simulink model "motor_simscapepump"  (R2014a)
settings: Solver=ode15s  StartTime=0.0  StopTime=1  MaxStep=0.2  RelTol=1e-4
undefined symbols (not defined in the file): D1, Delta
libraries: powerlib x6, fl_lib x4, nesl_utility x2, sh_lib x1
settings Model: Creator=scastro  LastModifiedBy=cosorio
settings DataIOCC: SaveOutput=off  SaveTime=off
settings DebuggingCC: UnderspecifiedInitializationDetection=Classic  MultiTaskDSMMsg=warning  MultiTaskCondExecSysMsg=none
settings RTWCC: IncludeERTFirstTime=on

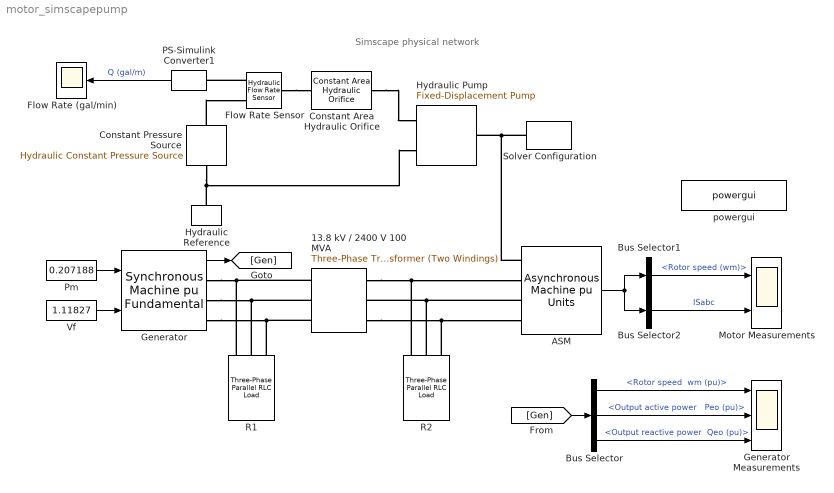
== system motor_simscapepump ==
  note: Simscape physical network
  13.8 kV / 2400 V 100 MVA : powerlib/Elements/Three-Phase Transformer (Two Windings)  Winding1Connection=Yg  UNITS=pu  NominalPower=[ 100e6 , 60 ]  Winding1=[ 13800 , 0.002 , 0.08 ]  Winding2Connection=Delta (D1)  Winding2=[ 2400 , 0.002 , 0.08 ]  SetSaturation=off  Rm=500  Lm=500  Saturation=[ 0,0 ; 0.0024,1.2 ; 1.0,1.52 ]  Hysteresis=off  DataFile='hysteresis'  SetInitialFlux=off  InitialFluxes=[ 0.8 , -0.8 , 0.7 ]  Measurements=None  MoreParameters=off  BreakLoop=off  DataType=off  TransfoNumber=1
  ASM : powerlib/Machines/Asynchronous Machine pu Units  PresetModel=No  MechanicalLoad=Mechanical rotational port  ShowDetailedParameters=on  RotorType=Squirrel-cage  ReferenceFrame=Rotor  Units=pu  MeasurementBus=off  NominalParameters=[10e6 2400 60]  Stator=[0.01965 0.0397]  Rotor=[0.01909 0.0397]  Cage1=[0.01909 0.0397]  Cage2=[0.01909 0.0397]  Lm=1.354  Mechanical=[0.09526 0.05479 2]  PolePairs=2  InitialConditions=[0.00133172 0 0.711213 0.711213 0.711213 -114.92 125.08 5.08024]  SimulateSaturation=off  Saturation="[0.212,0.4201,0.8125,1.0979,1.4799,2.2457,3.2586,4.5763,6.4763 ;   0.5,0.7,0.9,1,1.1,1.2 ,1.3,1.4,1.5]"  LoadFlowParameters=640000  TsPowergui=0  TsBlock=-1  IterativeModel=Trapezoidal non iterative  Pmec=25e6
      settings: AttributesFormatString=%<NominalParameters>
  Bus Selector : BusSelector  OutputSignals="Mechanical.Rotor speed  wm (pu),Output active power   Peo (pu),Output reactive power  Qeo (pu)"
  Bus Selector1 : BusSelector  OutputSignals=Mechanical.Rotor speed (wm)
  Bus Selector2 : BusSelector  OutputSignals=Stator measurements.Stator current is_a (pu),Stator measurements.Stator current is_b (pu),Stator measurements.Stator current is_c (pu)  OutputAsBus=on
  Constant Pressure Source : fl_lib/Hydraulic/Hydraulic Sources/Hydraulic Constant Pressure Source  commanded_pressure=50e5 Pa
      settings: AttributesFormatString=P = %<commanded_pressure> Pa
  Constant Area Hydraulic Orifice : fl_lib/Hydraulic/Hydraulic Elements/Constant Area Hydraulic Orifice  area=5e-4 m^2  C_d=0.7  Re_cr=12  D_h=0.0113 m  p_cr=1 Pa  q_specify=off  q_priority=High  q=1 m^3/s  p_specify=off  p_priority=High  p=0 Pa
  Flow Rate (gal/min) : Scope
      settings: YMin=0  YMax=300  SaveName=ScopeData4
  Flow Rate Sensor : fl_lib/Hydraulic/Hydraulic Sensors/Hydraulic Flow Rate Sensor
  Generator : powerlib/Machines/Synchronous Machine pu Fundamental  PresetModel=No  MechanicalLoad=Mechanical power Pm  ShowDetailedParameters=on  RotorType=Salient-pole  Units=per unit fundamental parameters  MeasurementBus=off  NominalParameters="[ 100E6  13800   60]"  Stator="[ 2.85E-03  0.114  1.19  0.36 ]"  Field="[ 5.79E-04  0.114]"  Dampers2=[0.0652, 0.5134, 0.0287, 0.2553, 7.765e-3, 0.9167 ]  Dampers1="[ 1.17E-02  0.182  1.97E-02  0.384 ]"  Mechanical=[ 3.7 0 2 ]  PolePairs=2  InitialConditions=[0 -84.5996 0.22005 0.22005 0.22005 -19.793 -139.793 100.207 1.11827]  SetSaturation=off  Saturation=[0.6404,0.7127,0.8441,0.9214,0.9956,1.082,1.19,1.316,1.457;0.7,0.7698,0.8872,0.9466,0.9969,1.046,1.1,1.151,1.201]  LoadFlowParameters=[2 75000000 13800 0 25000000]  TsPowergui=0  TsBlock=-1  IterativeModel=Trapezoidal non iterative  BusType=PQ  Pref=75e6  Qref=25e6  Qmin=-inf  Qmax=inf  PLF=0  QLF=0
      settings: AttributesFormatString=%<NominalParameters>
  Generator Measurements : Scope  NumInputPorts=3
      settings: YMin=0~0~0  YMax=1.5~1~1
  Hydraulic Pump : sh_lib/Pumps and Motors/Fixed-Displacement Pump  D=7.5e-5 m^3/rad  efficiency_vol=0.9  efficiency_tot=0.8  pr_nominal=100e5 Pa  w_nominal=60*2*pi rad/s  visc_nominal=18 cSt  dens_nominal=900 kg/m^3  k_leak=1e-11 m^3/s/Pa  efficiency_mech=0.7
  Hydraulic Reference : fl_lib/Hydraulic/Hydraulic Elements/Hydraulic Reference
  Motor Measurements : Scope  NumInputPorts=2
      settings: YMin=0~-1  YMax=1.5~1  SaveName=ScopeData2
  PS-Simulink Converter1 : nesl_utility/PS-Simulink Converter  PhysicalDomain=network_engine_domain  SubClassName=ps_output  LeftPortType=input  RightPortType=output  PseudoPeriodic=off  Frequencies=[]  Unit=gal/min  AffineConversion=off
  Pm : Constant  Value=0.207188
  R1 : powerlib/Elements/Three-Phase Parallel RLC Load  LConnTagsString=A|B|C  Configuration=Y (grounded)  NominalVoltage=13800  NominalFrequency=60  ActivePower=10e6  InductivePower=0  CapacitivePower=0  Measurements=None  LoadType=constant Z
      settings: AttributesFormatString=P = %<ActivePower>W
  R2 : powerlib/Elements/Three-Phase Parallel RLC Load  LConnTagsString=A|B|C  Configuration=Y (grounded)  NominalVoltage=2400  NominalFrequency=60  ActivePower=10e6  InductivePower=0  CapacitivePower=0  Measurements=None  LoadType=constant Z
      settings: AttributesFormatString=P = %<ActivePower>W
  Solver Configuration : nesl_utility/Solver Configuration  PhysicalDomain=network_engine_domain  SubClassName=solver  LeftPortType=input  RightPortType=generic  Accelerate=off  Tones=[]  Harmonics=[]  SimulateNoise=off  Profile=off  UseLocalSampling=off  EnableSwitchedLinearOptims=on  FrequencyDomain=off  UseCCode=off  RelTol=0.001  AbsTol=1e-06  MinStep=1e-09  ToWorkspace=off  DoDC=off  ResidualTolerance=1e-09  UseLocalSolver=off  LocalSolverChoice=NE_BACKWARD_EULER_ADVANCER  LocalSolverSampleTime=0.0001  DoFixedCost=off  MaxNonlinIter=3  MaxModeIter=2  LinearAlgebra=Sparse  DelaysMemoryBudget=1024  AutomaticFiltering=on  FilteringTimeConstant=0.001
  Vf : Constant  Value=1.11827
  powergui : powerlib/powergui  Priority=1  SimulationMode=Discrete  SolverType=Tustin  SampleTime=1e-4  frequency=60  SPID=off  DisableSnubberDevices=off  DisableRonSwitches=off  DisableVfSwitches=off  SwTol=0  Interpol=off  DisplayEquations=off  Ts=0  methode=off  frequencyindice=60  Pbase=100e6  ErrMax=0.0001  Iterations=50  UnitsV=kV  UnitsW=MW  FunctionMessages=off  echomessages=off  HookPort=off  EnableUseOfTLC=off  x0status=blocks  RestoreLinks=warning  ResistiveCurrentMeasurement=off  Frange=[0:2:500]  Ylog=off  Xlog=on  ShowGrid=off  save=off  variable=ZData  structure=0  ZoomFFT=off  StartTime=0.0  cycles=1  DisplayStyle=1  fundamental=60  FreqAxis=off  MaxFrequency=1000  frequencyindicesteady=1  RmsSteady=1  display=off
  wires:
  Bus Selector/3 -> Generator Measurements/3  "<Output reactive power  Qeo (pu)>"
  Bus Selector/2 -> Generator Measurements/2  "<Output active power   Peo (pu)>"
  Bus Selector/1 -> Generator Measurements/1  "<Rotor speed  wm (pu)>"
  ASM/1 -> Bus Selector1/1, Bus Selector2/1
  Bus Selector1/1 -> Motor Measurements/1  "<Rotor speed (wm)>"
  Vf/1 -> Generator/2
  Pm/1 -> Generator/1
  PS-Simulink Converter1/1 -> Flow Rate (gal/min)/1  "Q (gal/m)"
  Bus Selector2/1 -> Motor Measurements/2  "ISabc"
  Generator/1 -> [Gen]
  [Gen] -> Bus Selector/1
  connections:
  13.8 kV / 2400 V 100 MVA/LConn1 -- R1/LConn1 -- Generator/RConn1
  13.8 kV / 2400 V 100 MVA/LConn2 -- R1/LConn2 -- Generator/RConn2
  13.8 kV / 2400 V 100 MVA/LConn3 -- R1/LConn3 -- Generator/RConn3
  13.8 kV / 2400 V 100 MVA/RConn1 -- ASM/LConn2 -- R2/LConn1
  ASM/LConn3 -- R2/LConn2 -- 13.8 kV / 2400 V 100 MVA/RConn2
  13.8 kV / 2400 V 100 MVA/RConn3 -- ASM/LConn4 -- R2/LConn3
  Flow Rate Sensor/LConn1 -- Constant Area Hydraulic Orifice/RConn1
  Hydraulic Reference/LConn1 -- Constant Pressure Source/RConn1 -- Hydraulic Pump/RConn2
  Constant Area Hydraulic Orifice/LConn1 -- Hydraulic Pump/RConn1
  Flow Rate Sensor/RConn1 -- PS-Simulink Converter1/LConn1
  Constant Pressure Source/LConn1 -- Flow Rate Sensor/RConn2
  ASM/LConn1 -- Hydraulic Pump/LConn1 -- Solver Configuration/RConn1
